simulink model "lab1_system"  (R2024a)
settings: Solver=VariableStepAuto  StartTime=0.0  StopTime=40.0  FixedStep=1e-6  RelTol=1e-6
values from neighbouring files (symbols this model uses):
  a0 = 12    [untitled.m]
  a1 = 19    [untitled.m]
  a2 = 8    [untitled.m]
  b0 = 42    [untitled.m]
  b1 = 24    [untitled.m]
  b2 = 12    [untitled.m]
settings Model: Creator=alexivanov  LastModifiedBy=alexivanov

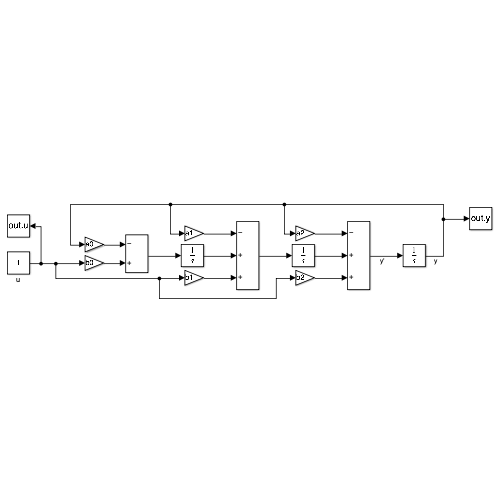
[thumbnail: Simulink's stored preview of the top-level diagram]
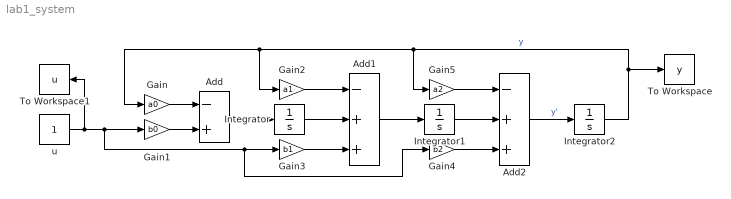
== system lab1_system ==
  Add : Sum  Inputs=-+
  Add1 : Sum  Inputs=-++
  Add2 : Sum  Inputs=-++
  Gain : Gain  Gain=a0
  Gain1 : Gain  Gain=b0
  Gain2 : Gain  Gain=a1
  Gain3 : Gain  Gain=b1
  Gain4 : Gain  Gain=b2
  Gain5 : Gain  Gain=a2
  Integrator : Integrator
  Integrator1 : Integrator
  Integrator2 : Integrator
  To Workspace : ToWorkspace  VariableName=y  SaveFormat=Timeseries  SampleTime=-1
  To Workspace1 : ToWorkspace  VariableName=u  SaveFormat=Timeseries  SampleTime=-1
  u : Constant  SampleTime=0
  wires:
  Gain/1 -> Add/1
  Gain1/1 -> Add/2
  Add/1 -> Integrator/1
  Integrator/1 -> Add1/2
  Gain2/1 -> Add1/1
  Gain3/1 -> Add1/3
  Add1/1 -> Integrator1/1
  Integrator1/1 -> Add2/2
  Gain5/1 -> Add2/1
  Gain4/1 -> Add2/3
  Add2/1 -> Integrator2/1  "y'"
  Integrator2/1 -> Gain2/1, Gain/1, Gain5/1, To Workspace/1  "y"
  u/1 -> To Workspace1/1, Gain4/1, Gain3/1, Gain1/1
